simulink model "MPC_Controller"  (R2019b)
settings: Solver=VariableStepAuto  StartTime=0.0  StopTime=simStopTime  RelTol=1e-3
values from neighbouring files (symbols this model uses):
  curvatures = [curvatures; mean([lb.Curvature])]    [helperCreateReferencePath.m]    (also in onStartup.m = evaluator.curvatures)
  directions = ones(size(speedProfile))    [ControllerScript.m]
  mass = 2500    [ControllerScript.m]
  refPoses = [refPoses; [egoVehicle.Position(1:2), egoVehicle.Yaw]]    [helperCreateReferencePath.m]
  s = getValuesToEstimate(Exp)    [parameterEstimation.m]
  speedProfile = sqrt(sum(speedVector.*speedVector,2))    [ControllerScript.m]    (also in extractTheData.m = evaluator.velocities)
  theta0 = refPoses(1, 3)    [helperCreateReferencePath.m]
  Ts = 0.1    [ControllerScript.m]
  VEH =     [VEH.mat]
  x0 = refPoses(1, 1)    [helperCreateReferencePath.m]
  y0 = refPoses(1, 2)    [helperCreateReferencePath.m]
undefined symbols (not defined in the file or in its folder): driving, speedVector
libraries: simulink x2, autolibshared x2, drivingscenarioandsensors x2, mpcadaslib x1, sim3dlib x1, sim3dautolib x1, vehdynlibviscommon x1
settings Model: EnablePacing=on  PacingRate=1000  OrderedModelArguments=off  Creator=alaa  LastModifiedBy=LapTime
settings DataIOCC: SaveOutput=off  SignalLogging=off  DSMLogging=off  SaveTime=off  OutputOption=AdditionalOutputTimes  OutputTimes=simStopTime  ReturnWorkspaceOutputsName=SDOSimTest_Log
settings DebuggingCC: AlgebraicLoopMsg=none  ArtificialAlgebraicLoopMsg=none  MaxConsecutiveZCsMsg=none  ParameterPrecisionLossMsg=none  OperatingPointInterfaceChecksumMismatchMsg=none

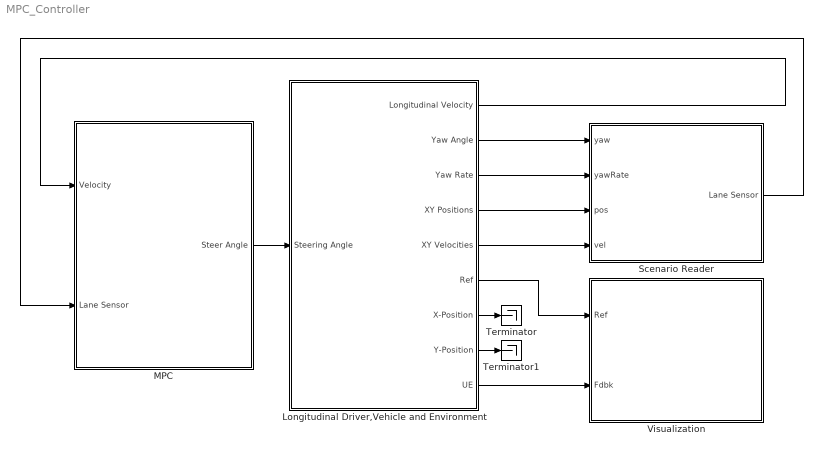
== system MPC_Controller ==
  Longitudinal Driver,Vehicle and Environment : Subsystem
  MPC : Subsystem
  Scenario Reader : Subsystem
  Terminator : Terminator
  Terminator1 : Terminator
  Visualization : Subsystem
  wires:
  Longitudinal Driver,Vehicle and Environment/1(Longitudinal Velocity) -> MPC/1(Velocity)
  Scenario Reader/1(Lane Sensor) -> MPC/2(Lane Sensor)
  Longitudinal Driver,Vehicle and Environment/5(XY Velocities) -> Scenario Reader/4(vel)
  Longitudinal Driver,Vehicle and Environment/2(Yaw Angle) -> Scenario Reader/1(yaw)
  Longitudinal Driver,Vehicle and Environment/3(Yaw Rate) -> Scenario Reader/2(yawRate)
  Longitudinal Driver,Vehicle and Environment/6(Ref) -> Visualization/1(Ref)
  Longitudinal Driver,Vehicle and Environment/4(XY Positions) -> Scenario Reader/3(pos)
  Longitudinal Driver,Vehicle and Environment/9("UE ") -> Visualization/2(Fdbk)
  Longitudinal Driver,Vehicle and Environment/7(X-Position) -> Terminator/1
  Longitudinal Driver,Vehicle and Environment/8(Y-Position) -> Terminator1/1
  MPC/1(Steer Angle) -> Longitudinal Driver,Vehicle and Environment/1(Steering Angle)

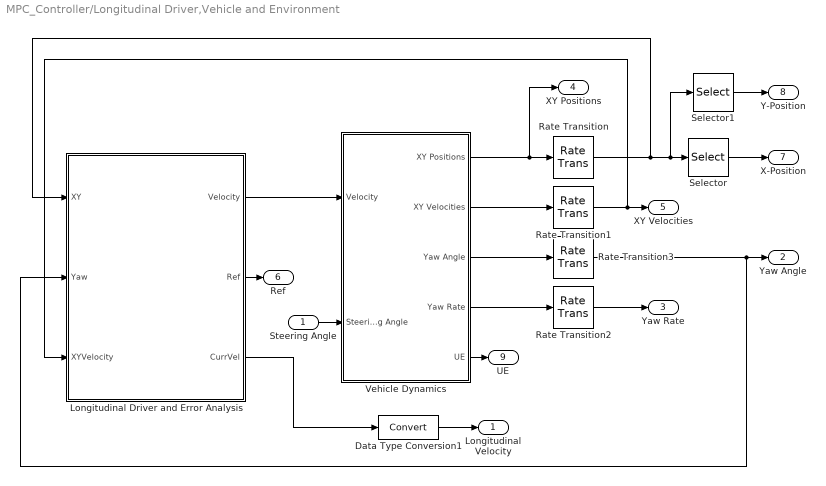
== system MPC_Controller/Longitudinal Driver,Vehicle and Environment ==
  Steering Angle : Inport  Unit=rad
  Data Type Conversion1 : DataTypeConversion
  Longitudinal Driver and Error Analysis : Subsystem
  Rate Transition : RateTransition  InitialCondition=[x0,y0]  OutPortSampleTime=Ts
  Rate Transition1 : RateTransition  InitialCondition=speedVector(1,1:2)  OutPortSampleTime=Ts
  Rate Transition2 : RateTransition  OutPortSampleTime=Ts
  Rate Transition3 : RateTransition  OutPortSampleTime=Ts
  Selector : Selector  InputPortWidth=2  IndexOptions=Index vector (dialog)  Indices=[1]  OutputSizes=1
  Selector1 : Selector  InputPortWidth=2  IndexOptions=Index vector (dialog)  Indices=[2]  OutputSizes=1
  Vehicle Dynamics : Subsystem  VariantControl=VariantVDBS
  Longitudinal Velocity : Outport  OutDataTypeStr=single  Unit=m/s  VectorParamsAs1DForOutWhenUnconnected=off
  Yaw Angle : Outport  Port=2
  Yaw Rate : Outport  Port=3
  XY Positions : Outport  Port=4
  XY Velocities : Outport  Port=5
  Ref : Outport  Port=6
  X-Position : Outport  Port=7
  Y-Position : Outport  Port=8
  "UE " : Outport  Port=9
  wires:
  Vehicle Dynamics/3(Yaw Angle) -> Rate Transition3/1
  Steering Angle/1 -> Vehicle Dynamics/2(Steering Angle)
  Data Type Conversion1/1 -> Longitudinal Velocity/1
  Longitudinal Driver and Error Analysis/3(CurrVel) -> Data Type Conversion1/1
  Longitudinal Driver and Error Analysis/1(Velocity) -> Vehicle Dynamics/1(Velocity)
  Selector/1 -> X-Position/1
  Selector1/1 -> Y-Position/1
  Vehicle Dynamics/2(XY Velocities) -> Rate Transition1/1
  Vehicle Dynamics/4(Yaw Rate) -> Rate Transition2/1
  Longitudinal Driver and Error Analysis/2(Ref) -> Ref/1
  Vehicle Dynamics/5("UE ") -> "UE "/1
  Rate Transition2/1 -> Yaw Rate/1
  Rate Transition1/1 -> XY Velocities/1, Longitudinal Driver and Error Analysis/3(XYVelocity)
  Rate Transition3/1 -> Yaw Angle/1, Longitudinal Driver and Error Analysis/2(Yaw)
  Vehicle Dynamics/1(XY Positions) -> XY Positions/1, Rate Transition/1
  Rate Transition/1 -> Selector1/1, Selector/1, Longitudinal Driver and Error Analysis/1(XY)

== system MPC_Controller/MPC ==
  Velocity : Inport
  Lane Sensor : Inport  Port=2
  Lane Center : Subsystem
  Lane Keeping Controller : mpcadaslib/Lane Keeping Assist System  ModelType=Use vehicle parameters  VehicleMass=mass  VehicleYawInertia=VEH.YawMomentInertia  LengthToFront=wheelbase-drear  LengthToRear=wheelbase-dfront  FrontTireStiffness=f_tire_stiff  RearTireStiffness=r_tire_stiff  EgoModelMatrixA=[-4.4021 ,-12.4603;1.3913,-5.1868]  EgoModelMatrixB=[24.1270;15.8609]  EgoModelMatrixC=[1,0;0,1]  InitialLongVel=speedProfile(1)  TransportLag=0  MinSteering=min_steer  umin_ext=off  MaxSteering=max_steer  umax_ext=off  Ts=Ts  PredictionHorizon=pred_Horizon  ControllerBehavior=aggressive  suboptimal=off  maxiter=10  datatypeopt=single  optmode=off  trackmode=off
      settings: SourceProductName=Model Predictive Control Toolbox  SourceProductBaseCode=MP
  Steer Angle : Outport
  wires:
  Lane Center/3(Heading Angle) -> Lane Keeping Controller/4
  Velocity/1 -> Lane Keeping Controller/2, Lane Center/2(Longitudinal Velocity)
  Lane Center/1(Previewed Curvature) -> Lane Keeping Controller/1
  Lane Center/2(Lateral Offset) -> Lane Keeping Controller/3
  Lane Sensor/1 -> Lane Center/1(Lane Detections)
  Lane Keeping Controller/1 -> Steer Angle/1

== system MPC_Controller/Scenario Reader ==
  yaw : Inport
  yawRate : Inport  Port=2
  pos : Inport  Port=3
  vel : Inport  Port=4
  Pack Ego Actor1 : MATLAB Function  TreatAsAtomicUnit=on
  Pack to Custom Sensor Data Format : Subsystem
  Scenario Reader : drivingscenarioandsensors/Scenario Reader  ScenarioSource=From workspace  ScenarioFileName=/home/alaa/Downloads/race-track-optimization/inc/controller/ankit.mat  ScenarioVariableName=scenario  OutputCoordinateSystem=Vehicle coordinates  EgoVehicleSource=Input port  EgoVehicleActorID=1  SampleTime=Ts  LaneBoundaryOutput=Ego vehicle lane boundaries  LaneBoundaryDistance=0:0.5:60  LaneBoundaryLocation=Inner edge of lane markings  BusNameSource=Auto  BusName=BusActors1Actors  BusName2Source=Auto  BusName2=BusLaneBoundaries  SimulateUsing=Interpreted execution
      settings: SourceProductName=Automated Driving Toolbox
  Terminator : Terminator
  Vision Detection Generator : drivingscenarioandsensors/Vision Detection Generator  SensorIndex=1  DetectorOutput=Lanes only  UpdateInterval=0.1  LaneUpdateInterval=0.1  SensorLocation=[ 1.9, 0 ]  Height=1.1  Yaw=0  Pitch=1  Roll=0  BusNameSource=Auto  BusName=BusObjectDetections  BusName2Source=Auto  BusName2=BusVision  MaxNumDetectionsSource=Property  MaxNumDetections=50  MaxNumLanesSource=Property  MaxNumLanes=2  DetectionCoordinates=Ego Cartesian  SimulateUsing=Interpreted execution  MaxRange=150  BoundingBoxAccuracy=5  ProcessNoiseIntensity=5  MaxSpeed=50  MaxAllowedOcclusion=0.5  MinObjectImageSize=[ 15, 15 ]  DetectionProbability=0.9  FalsePositivesPerImage=0.1  MinLaneImageSize=[ 20, 3 ]  LaneBoundaryAccuracy=3  HasNoise=on  InitialSeedSource=Repeatable  InitialSeed=0  UsedSeed=driving.internal.SimulinkUtilities.seedManager(gcb)  ActorProfilesSource=Parameters  ActorProfilesParameters=driving.internal.ActorProfilesParameters  ActorProfilesExpression=struct( 'ClassID', 0, 'Length', 4.7, 'Width', 1.8, 'Height', 1.4, 'OriginOffset', [ -1.35, 0, 0 ] )  Intrinsics=driving.internal.cameraIntrinsics
      settings: SourceProductName=Automated Driving Toolbox
  Lane Sensor : Outport
  wires:
  Pack Ego Actor1/1(a) -> Scenario Reader/1
  pos/1 -> Pack Ego Actor1/1(pos)
  Pack to Custom Sensor Data Format/1(Out) -> Lane Sensor/1
  Scenario Reader/2 -> Vision Detection Generator/1
  yaw/1 -> Pack Ego Actor1/3(yaw)
  Scenario Reader/1 -> Terminator/1
  Vision Detection Generator/1 -> Pack to Custom Sensor Data Format/1(In)
  vel/1 -> Pack Ego Actor1/2(vel)
  yawRate/1 -> Pack Ego Actor1/4(yawRate)

== system MPC_Controller/Visualization ==
  Ref : Inport
  Fdbk : Inport  Port=2
  Bus Selector : BusSelector  OutputSignals=InertFrm.Cg.Disp.X,InertFrm.Cg.Disp.Y,InertFrm.Cg.Vel.Xdot,InertFrm.Cg.Vel.Ydot
  Bus Selector1 : BusSelector  OutputSignals=InertFrm.Cg.Ang.phi,InertFrm.Cg.Ang.theta,InertFrm.Cg.Ang.psi  OutputAsBus=on
  Bus Selector5 : BusSelector  OutputSignals=BdyFrm.FrntAxl.Steer.WhlAngFR,BdyFrm.FrntAxl.Steer.WhlAngFL,BdyFrm.RearAxl.Steer.WhlAngRR,BdyFrm.RearAxl.Steer.WhlAngRL  OutputAsBus=on
  Bus to Vector1 : BusToVector
  Bus to Vector2 : BusToVector
  Mux : Mux  Inputs=2
  Mux1 : Mux  Inputs=2
  UE : Subsystem  Commented=on
  Visualization : Subsystem
  wires:
  Mux/1 -> Visualization/1(position)
  Mux1/1 -> Visualization/2(Velocity)
  Bus to Vector1/1 -> Visualization/5(WhlAng)
  Ref/1 -> Visualization/3(Ref)
  Bus to Vector2/1 -> Visualization/4(InertAng)
  Bus Selector/3 -> Mux1/1  "<Xdot>"
  Bus Selector/4 -> Mux1/2  "<Ydot>"
  Bus Selector/2 -> Mux/2  "<Y>"
  Bus Selector/1 -> Mux/1  "<X>"
  Fdbk/1 -> UE/1(VehFdbk), Bus Selector5/1, Bus Selector1/1, Bus Selector/1
  Bus Selector5/1 -> Bus to Vector1/1
  Bus Selector1/1 -> Bus to Vector2/1

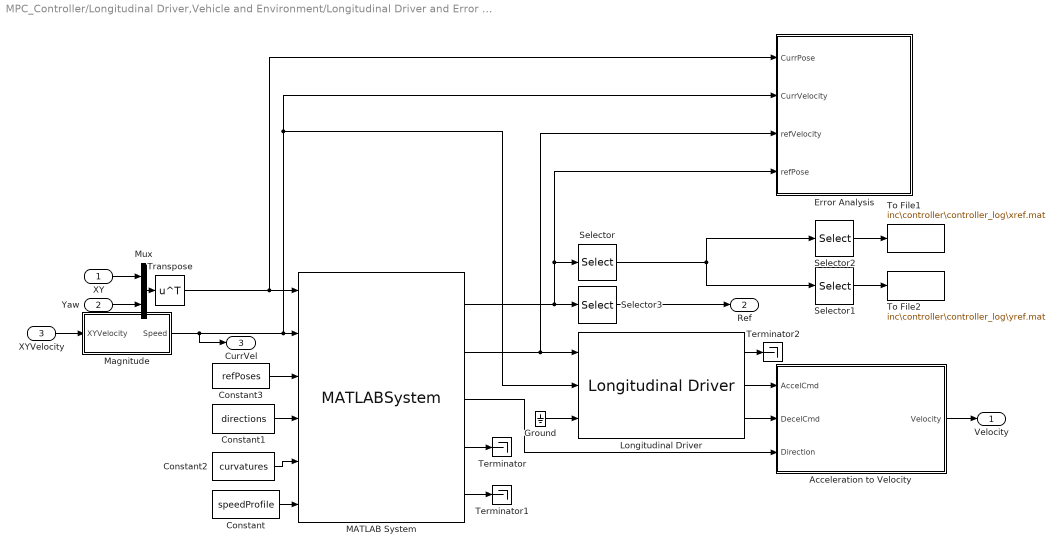
== system MPC_Controller/Longitudinal Driver,Vehicle and Environment/Longitudinal Driver and Error Analysis ==
  XY : Inport
  Yaw : Inport  Port=2
  XYVelocity : Inport  Port=3
  Acceleration to Velocity : Subsystem  TreatAsAtomicUnit=on
  Constant : Constant  Value=speedProfile  SampleTime=Ts
  Constant1 : Constant  Value=directions  SampleTime=Ts
  Constant2 : Constant  Value=curvatures  SampleTime=Ts
  Constant3 : Constant  Value=refPoses  SampleTime=Ts
  Error Analysis : Subsystem
  Ground : Ground
  Longitudinal Driver : autolibshared/Longitudinal Driver  cntrlType=Predictive  shftType=None  velUnits=m/s  gearOut=off  Kp=5  Ki=5  Kff=.1  Kg=0  VehVelVec=[0 100]  KffVec=[.1 .1]  KpVec=[10 10]  KiVec=[5 5]  KgVec=[0 0]  m=mass  Kpt=3000  tau=0.01  L=5  aR=200  bR=2.5  cR=VEH.DragCoefficient  g=9.81  vnom=5  Kaw=1  tauerr=.01  tauPt=2  GearInit=0  tShift=.1  pdlVec=[0.1 0.4 0.5 0.9]  upShftTbl=[-1 12.9375 26.4375 39.9375 51.18749999999999 62.4375 72.84375 83.25;-1 16.3125 29.8125 43.3125 54.5624 65.8125 76.78125 87.75;-1 19.6875 33.1875 46.68749999999999 57.9375 69.1875 80.71875 92.25;-1 33 52.5 77.25 100.5 138.75 161.875 185]  dwnShftTbl=[1 9.5625 23.0625 36.5625 47.8125 59.0625 68.90625 78.75;1 12.9375 26.4375 39.9375 51.18749999999999 62.4375 72.84375 83.25;1 16.3125 29.8125 43.3125 54.562499 65.8125 76.78125 87.75;1 19.6875 33.1875 46.68749999999999 57.9375 69.1875 80.71875 92.25]  tClutch=.5  tRev=.5  tPark=120  aMode=2  UpGearVec="[0  1  2  3  4  5  6  7]"  DownGearVec="[1  2  3  4  5  6  7  8]"
      settings: SourceProductName=Powertrain Blockset  SourceProductBaseCode=PW
  MATLAB System : MATLABSystem  System=HelperPathAnalyzer  Wheelbase=wheelbase  HasResetOutput=on  SimulateUsing=Interpreted execution
      mask Type: HelperPathAnalyzer
      mask Display:
      | disp(['Helper' char(10) 'Path' char(10) 'Analyzer']);
      | port_label('input',1,'CurrPose');
      | port_label('input',2,'CurrVelocity');
      | port_label('input',3,'RefPoses');
      | port_label('input',4,'Directions');
      | port_label('input',5,'Curvatures');
      | port_label('input',6,'SpeedProfile');
      | port_label('output',1,'RefPose');
      | port_label('output',2,'RefVelocity');
      | port_label('output',3,'Direction');
      | port_label('output',4,'Curvature');
      | port_label('output',5,'Reset');
  Magnitude : Subsystem
  Mux : Mux  Inputs=2
  Selector : Selector  InputPortWidth=3  IndexOptions=Index vector (dialog)  Indices=[1 2]  OutputSizes=1
  Selector1 : Selector  InputPortWidth=2  IndexOptions=Index vector (dialog)  Indices=[2]  OutputSizes=1
  Selector2 : Selector  InputPortWidth=2  IndexOptions=Index vector (dialog)  Indices=[1]  OutputSizes=1
  Selector3 : Selector  InputPortWidth=3  IndexOptions=Index vector (dialog)  Indices=[1 2]  OutputSizes=1
  Terminator : Terminator
  Terminator1 : Terminator
  Terminator2 : Terminator
  To File1 : ToFile  Filename=inc\controller\controller_log\xref.mat  MatrixName=xref
  To File2 : ToFile  Filename=inc\controller\controller_log\yref.mat  MatrixName=yref
  Transpose : Math  Operator=transpose  SignedPower=off  SaturateOnIntegerOverflow=on
  Velocity : Outport
  Ref : Outport  Port=2
  CurrVel : Outport  Port=3
  wires:
  MATLAB System/2 -> Error Analysis/3(refVelocity), Longitudinal Driver/1
  Constant2/1 -> MATLAB System/5
  Mux/1 -> Transpose/1
  Acceleration to Velocity/1(Velocity) -> Velocity/1
  Constant1/1 -> MATLAB System/4
  Constant/1 -> MATLAB System/6
  XY/1 -> Mux/1
  Selector/1 -> Selector2/1, Selector1/1
  MATLAB System/3 -> Acceleration to Velocity/3(Direction)
  Magnitude/1(Speed) -> CurrVel/1, Error Analysis/2(CurrVelocity), Longitudinal Driver/2, MATLAB System/2
  XYVelocity/1 -> Magnitude/1(XYVelocity)
  Yaw/1 -> Mux/2
  Longitudinal Driver/3 -> Acceleration to Velocity/2(DecelCmd)
  Longitudinal Driver/2 -> Acceleration to Velocity/1(AccelCmd)
  Selector2/1 -> To File1/1
  Selector1/1 -> To File2/1
  Constant3/1 -> MATLAB System/3
  MATLAB System/1 -> Selector3/1, Selector/1, Error Analysis/4(refPose)
  MATLAB System/5 -> Terminator1/1
  MATLAB System/4 -> Terminator/1
  Longitudinal Driver/1 -> Terminator2/1
  Ground/1 -> Longitudinal Driver/3
  Selector3/1 -> Ref/1
  Transpose/1 -> MATLAB System/1, Error Analysis/1(CurrPose)

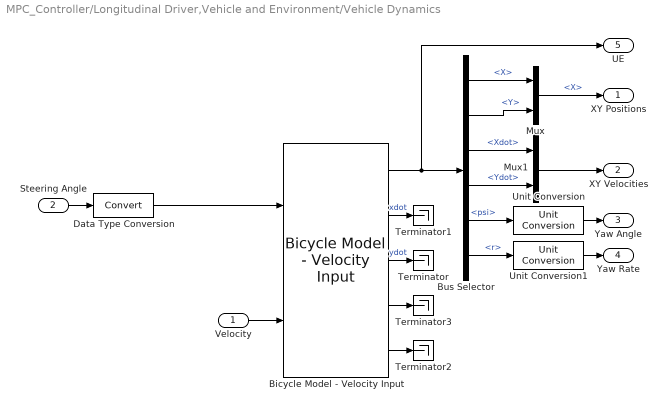
== system MPC_Controller/Longitudinal Driver,Vehicle and Environment/Vehicle Dynamics ==
  Velocity : Inport
  Steering Angle : Inport  Port=2
  Bicycle Model - Velocity Input : autolibshared/Bicycle Model - Velocity Input  trackMode=Single (bicycle)  inputMode=External longitudinal forces  frontSteerMode=on  rearSteerMode=off  windMode=off  muMode=off  extFMode=off  extMMode=off  aMode=3  NF=2  NR=2  m=mass  a=wheelbase-drear  b=wheelbase-dfront  h=h  X_o=x0  xdot_o=0  CalphaMode=off  sigmaMode=on  w=[1.4,1.4]  Cy_f=f_tire_stiff  Cy_r=r_tire_stiff  sigma_f=.1  sigma_r=.1  alpha_f_brk=[-.1 .1]  Cy_f_data=[-9e3 9e3]  alpha_r_brk=[-.1 .1]  Cy_r_data=[-9e3 9e3]  Y_o=y0  ydot_o=speedVector(1,2)  Izz=VEH.YawMomentInertia  psi_o=theta0*pi/180  r_o=0  Af=VEH.FrontalArea  Cd=VEH.DragCoefficient  Cl=0.1  Cpm=.1  beta_w=[0:0.01:0.3]  Cs=[0:0.03:0.9]  Cym=[0:0.01:0.3]  Pabs=101325  Tair=273  g=9.81  mu=mu  xdot_tol=.01  Fznom=5000  Fxtire_sat=1e6  Fytire_sat=1e6  longOff=0  latOff=0  vertOff=0
      settings: SourceProductName=Powertrain Blockset  SourceProductBaseCode=PW
  Bus Selector : BusSelector  OutputSignals=InertFrm.Cg.Disp.X,InertFrm.Cg.Disp.Y,InertFrm.Cg.Vel.Xdot,InertFrm.Cg.Vel.Ydot,InertFrm.Cg.Ang.psi,BdyFrm.Cg.AngVel.r
  Data Type Conversion : DataTypeConversion
  Mux : Mux  Inputs=2
  Mux1 : Mux  Inputs=2
  Terminator{,1..3} (4 alike) : Terminator
  Unit Conversion : UnitConversion  OutputType=Inherit: Inherit via back propagation
  Unit Conversion1 : UnitConversion  OutputType=Inherit: Inherit via back propagation
  XY Positions : Outport  Unit=m  VectorParamsAs1DForOutWhenUnconnected=off
  XY Velocities : Outport  Port=2  Unit=m/s  VectorParamsAs1DForOutWhenUnconnected=off
  Yaw Angle : Outport  Port=3  Unit=deg  VectorParamsAs1DForOutWhenUnconnected=off
  Yaw Rate : Outport  Port=4  Unit=degree/s  VectorParamsAs1DForOutWhenUnconnected=off
  "UE " : Outport  Port=5
  wires:
  Mux1/1 -> XY Velocities/1
  Unit Conversion1/1 -> Yaw Rate/1
  Unit Conversion/1 -> Yaw Angle/1
  Bus Selector/1 -> Mux/1  "<X>"
  Bus Selector/2 -> Mux/2  "<Y>"
  Bus Selector/4 -> Mux1/2  "<Ydot>"
  Bus Selector/3 -> Mux1/1  "<Xdot>"
  Steering Angle/1 -> Data Type Conversion/1
  Data Type Conversion/1 -> Bicycle Model - Velocity Input/1
  Velocity/1 -> Bicycle Model - Velocity Input/2
  Mux/1 -> XY Positions/1  "<X>"
  Bicycle Model - Velocity Input/1 -> "UE "/1, Bus Selector/1
  Bicycle Model - Velocity Input/2 -> Terminator1/1  "xdot"
  Bicycle Model - Velocity Input/3 -> Terminator/1  "ydot"
  Bus Selector/5 -> Unit Conversion/1  "<psi>"
  Bus Selector/6 -> Unit Conversion1/1  "<r>"
  Bicycle Model - Velocity Input/5 -> Terminator2/1
  Bicycle Model - Velocity Input/4 -> Terminator3/1

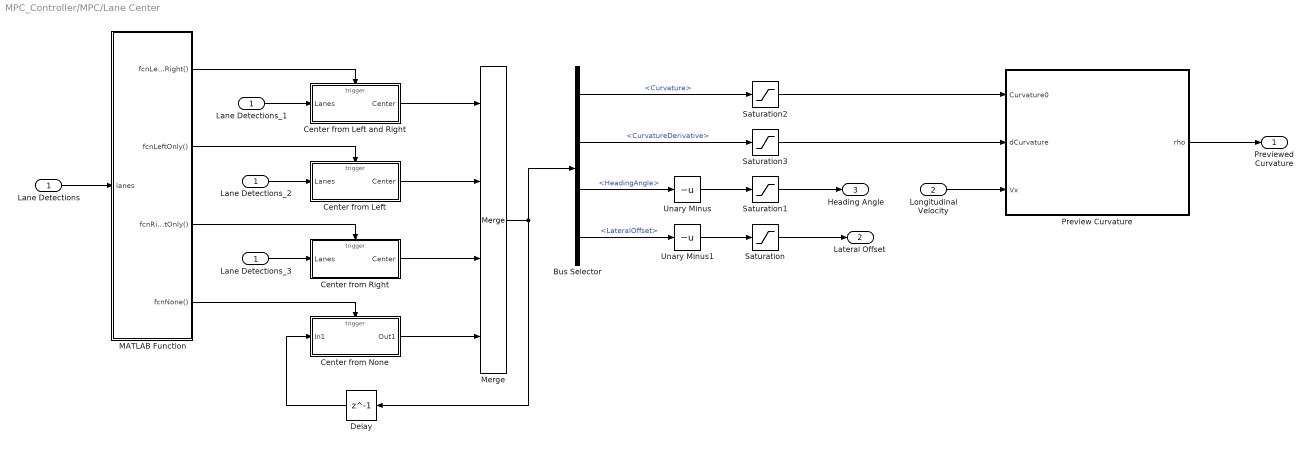
== system MPC_Controller/MPC/Lane Center ==
  Lane Detections : Inport
  Longitudinal Velocity : Inport  Port=2  OutDataTypeStr=single
  Bus Selector : BusSelector  OutputSignals=Curvature,CurvatureDerivative,HeadingAngle,LateralOffset
  Center from Left : Subsystem  TreatAsAtomicUnit=on
  Center from Left and Right : Subsystem  TreatAsAtomicUnit=on
  Center from None : Subsystem  TreatAsAtomicUnit=on
  Center from Right : Subsystem  TreatAsAtomicUnit=on
  Delay : Delay  DelayLength=1
  Lane Detections_1 : InportShadow
  Lane Detections_2 : InportShadow
  Lane Detections_3 : InportShadow
  MATLAB Function : MATLAB Function  TreatAsAtomicUnit=on
  Merge : Merge  Inputs=4
  Preview Curvature : MATLAB Function  TreatAsAtomicUnit=on  SystemSampleTime=Ts
  Saturation : Saturate
  Saturation1 : Saturate  UpperLimit=0.6  LowerLimit=-0.6
  Saturation2 : Saturate  UpperLimit=0.15  LowerLimit=-0.15
  Saturation3 : Saturate  UpperLimit=0.06  LowerLimit=-0.06
  Unary Minus : UnaryMinus
  Unary Minus1 : UnaryMinus
  Previewed Curvature : Outport  VectorParamsAs1DForOutWhenUnconnected=off
  Lateral Offset : Outport  Port=2  VectorParamsAs1DForOutWhenUnconnected=off
  Heading Angle : Outport  Port=3  VectorParamsAs1DForOutWhenUnconnected=off
  wires:
  Saturation2/1 -> Preview Curvature/1(Curvature0)
  Bus Selector/2 -> Saturation3/1  "<CurvatureDerivative>"
  Longitudinal Velocity/1 -> Preview Curvature/3(Vx)
  Merge/1 -> Delay/1, Bus Selector/1
  Center from Left and Right/1(Center) -> Merge/1
  Unary Minus/1 -> Saturation1/1
  Center from None/1(Out1) -> Merge/4
  MATLAB Function/3(fcnRightOnly()) -> Center from Right/Trigger
  Lane Detections_2/1 -> Center from Left/1(Lanes)
  MATLAB Function/1(fcnLeftAndRight()) -> Center from Left and Right/Trigger
  MATLAB Function/2(fcnLeftOnly()) -> Center from Left/Trigger
  Preview Curvature/1(rho) -> Previewed Curvature/1
  Saturation/1 -> Lateral Offset/1
  Lane Detections_1/1 -> Center from Left and Right/1(Lanes)
  Lane Detections/1 -> MATLAB Function/1(lanes)
  Bus Selector/1 -> Saturation2/1  "<Curvature>"
  Center from Right/1(Center) -> Merge/3
  Saturation1/1 -> Heading Angle/1
  Saturation3/1 -> Preview Curvature/2(dCurvature)
  Center from Left/1(Center) -> Merge/2
  Bus Selector/4 -> Unary Minus1/1  "<LateralOffset>"
  Delay/1 -> Center from None/1(In1)
  Unary Minus1/1 -> Saturation/1
  Bus Selector/3 -> Unary Minus/1  "<HeadingAngle>"
  Lane Detections_3/1 -> Center from Right/1(Lanes)
  MATLAB Function/4(fcnNone()) -> Center from None/Trigger

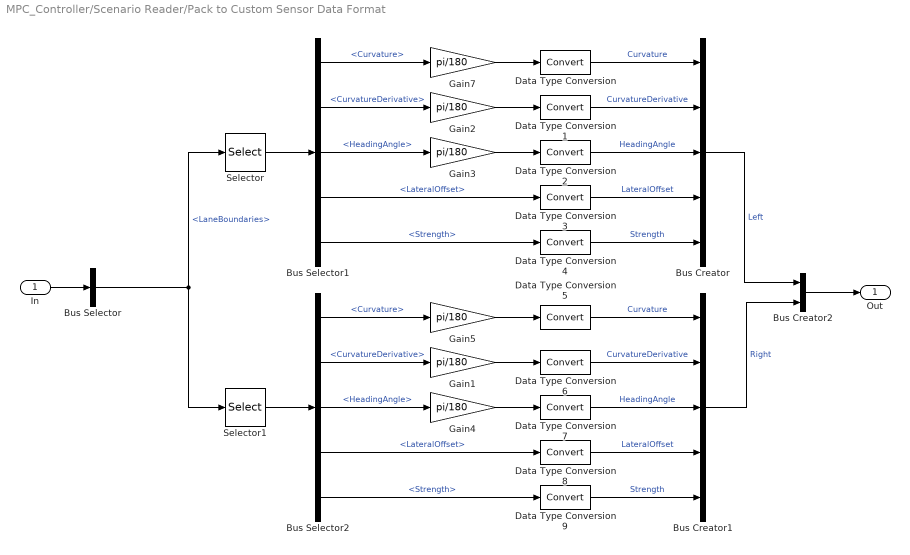
== system MPC_Controller/Scenario Reader/Pack to Custom Sensor Data Format ==
  In : Inport
  Bus Creator : BusCreator  Inputs=5  OutDataTypeStr=Bus: LaneSensorBoundaries
      settings: InheritFromInputs=off
  Bus Creator1 : BusCreator  Inputs=5  OutDataTypeStr=Bus: LaneSensorBoundaries
  Bus Creator2 : BusCreator  Inputs=2  OutDataTypeStr=Bus: LaneSensor
  Bus Selector : BusSelector  OutputSignals=LaneBoundaries
  Bus Selector1 : BusSelector  OutputSignals=Curvature,CurvatureDerivative,HeadingAngle,LateralOffset,Strength
  Bus Selector2 : BusSelector  OutputSignals=Curvature,CurvatureDerivative,HeadingAngle,LateralOffset,Strength
  Data Type Conversion{,1..9} (10 alike) : DataTypeConversion
  Gain{1..5,7} (6 alike) : Gain  Gain=pi/180
  Selector : Selector  InputPortWidth=2  IndexOptions=Index vector (dialog)  Indices=1  OutputSizes=1
  Selector1 : Selector  InputPortWidth=2  IndexOptions=Index vector (dialog)  Indices=2  OutputSizes=1
  Out : Outport  VectorParamsAs1DForOutWhenUnconnected=off
  wires:
  In/1 -> Bus Selector/1
  Bus Selector/1 -> Selector/1, Selector1/1  "<LaneBoundaries>"
  Selector/1 -> Bus Selector1/1
  Bus Selector1/2 -> Gain2/1  "<CurvatureDerivative>"
  Bus Selector1/1 -> Gain7/1  "<Curvature>"
  Bus Selector1/3 -> Gain3/1  "<HeadingAngle>"
  Gain7/1 -> Data Type Conversion/1
  Gain2/1 -> Data Type Conversion1/1
  Gain3/1 -> Data Type Conversion2/1
  Bus Selector1/4 -> Data Type Conversion3/1  "<LateralOffset>"
  Bus Selector1/5 -> Data Type Conversion4/1  "<Strength>"
  Data Type Conversion/1 -> Bus Creator/1  "Curvature"
  Data Type Conversion1/1 -> Bus Creator/2  "CurvatureDerivative"
  Data Type Conversion2/1 -> Bus Creator/3  "HeadingAngle"
  Data Type Conversion3/1 -> Bus Creator/4  "LateralOffset"
  Data Type Conversion4/1 -> Bus Creator/5  "Strength"
  Data Type Conversion9/1 -> Bus Creator1/5  "Strength"
  Data Type Conversion6/1 -> Bus Creator1/2  "CurvatureDerivative"
  Data Type Conversion7/1 -> Bus Creator1/3  "HeadingAngle"
  Data Type Conversion8/1 -> Bus Creator1/4  "LateralOffset"
  Data Type Conversion5/1 -> Bus Creator1/1  "Curvature"
  Bus Selector2/1 -> Gain5/1  "<Curvature>"
  Selector1/1 -> Bus Selector2/1
  Bus Selector2/4 -> Data Type Conversion8/1  "<LateralOffset>"
  Bus Selector2/5 -> Data Type Conversion9/1  "<Strength>"
  Bus Selector2/2 -> Gain1/1  "<CurvatureDerivative>"
  Gain4/1 -> Data Type Conversion7/1
  Gain5/1 -> Data Type Conversion5/1
  Gain1/1 -> Data Type Conversion6/1
  Bus Selector2/3 -> Gain4/1  "<HeadingAngle>"
  Bus Creator2/1 -> Out/1
  Bus Creator/1 -> Bus Creator2/1  "Left"
  Bus Creator1/1 -> Bus Creator2/2  "Right"

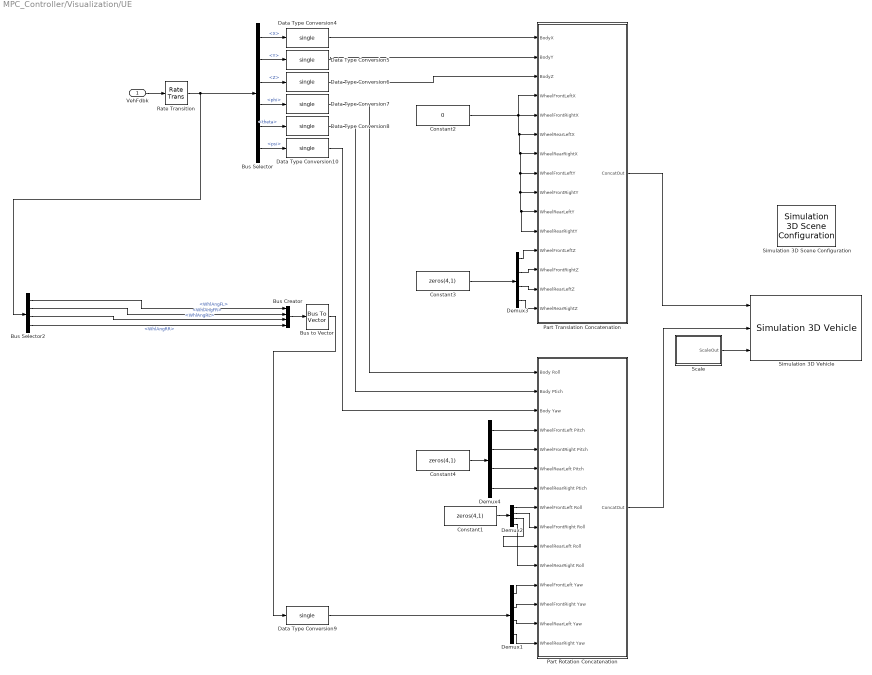
== system MPC_Controller/Visualization/UE ==
  VehFdbk : Inport
  Bus Creator : BusCreator  Inputs=4
  Bus Selector : BusSelector  OutputSignals=InertFrm.Cg.Disp.X,InertFrm.Cg.Disp.Y,InertFrm.Cg.Disp.Z,InertFrm.Cg.Ang.phi,InertFrm.Cg.Ang.theta,InertFrm.Cg.Ang.psi
  Bus Selector2 : BusSelector  OutputSignals=BdyFrm.FrntAxl.Steer.WhlAngFL,BdyFrm.FrntAxl.Steer.WhlAngFR,BdyFrm.RearAxl.Steer.WhlAngRL,BdyFrm.RearAxl.Steer.WhlAngRR
  Bus to Vector : BusToVector
  Constant1 : Constant  Value=zeros(4,1)  OutDataTypeStr=single
  Constant2 : Constant  Value=0  OutDataTypeStr=single
  Constant3 : Constant  Value=zeros(4,1)  OutDataTypeStr=single
  Constant4 : Constant  Value=zeros(4,1)  OutDataTypeStr=single
  Data Type Conversion{4..10} (7 alike) : DataTypeConversion  OutDataTypeStr=single
  Demux{1..4} (4 alike) : Demux
  Part Rotation Concatenation : Subsystem
  Part Translation Concatenation : Subsystem
  Rate Transition : RateTransition  OutPortSampleTime=Ts
  Scale : Subsystem
  Simulation 3D Scene Configuration : sim3dlib/Simulation 3D Scene Configuration  Priority=0  SceneDesc=US city block  vehTagList={'Scene Origin';'SimulinkVehicle1'}  vehTag=SimulinkVehicle1  OpVisEn=off  Ts=Ts  ProjectFormat=Executable  ProjectName=VehicleSimulation.exe  sensorTag=MainCamera1  sensorId=1  sensorName=MainCamera1  mountLoc=Origin  offsetFlag=off  tmountOffset=[0, 0, 0]  rmountOffset=[0, 0, 0]  HorizontalResolution=1280  VerticalResolution=720  HorizontalFOV=60  mountPoint=[0 0 0]  mountOrientation=[0 0 0]  aMode=aMode  ID=1
      settings: SourceProductName=Automated Driving Toolbox  SourceProductBaseCode=DR
  Simulation 3D Vehicle : sim3dautolib/Simulation 3D Vehicle  Priority=-1  PassVehMesh=Muscle car  VehColor=Red  ActorName=SimulinkVehicle1  Translation=[x0 y0 0; 0 0 0; 0 0 0; 0 0 0; 0 0 0]  Rotation=[0 0 theta0; 0 0 0; 0 0 0; 0 0 0; 0 0 0]  Scale=ones( 5, 3 )  SampleTime=Ts  ActorType=SimulinkVehicle  ID=1  aMode=2  ActorTag=SimulinkVehicle1
      settings: SourceProductName=Automated Driving Toolbox  SourceProductBaseCode=DR
  wires:
  Demux2/2 -> Part Rotation Concatenation/9(WheelFrontRight Roll)
  Bus Selector/5 -> Data Type Conversion8/1  "<theta>"
  Demux2/1 -> Part Rotation Concatenation/8(WheelFrontLeft Roll)
  Data Type Conversion6/1 -> Part Translation Concatenation/3(BodyZ)
  Demux1/4 -> Part Rotation Concatenation/15(WheelRearRight Yaw)
  Bus Selector/3 -> Data Type Conversion6/1  "<Z>"
  Data Type Conversion9/1 -> Demux1/1
  Data Type Conversion7/1 -> Part Rotation Concatenation/1(Body Roll)
  Rate Transition/1 -> Bus Selector/1, Bus Selector2/1
  Bus Selector/6 -> Data Type Conversion10/1  "<psi>"
  Demux2/3 -> Part Rotation Concatenation/10(WheelRearLeft Roll)
  Data Type Conversion4/1 -> Part Translation Concatenation/1(BodyX)
  Constant2/1 -> Part Translation Concatenation/5(WheelFrontRightX), Part Translation Concatenation/6(WheelRearLeftX), Part Translation Concatenation/7(WheelRearRightX), Part Translation Concatenation/8(WheelFrontLeftY), Part Translation Concatenation/9(WheelFrontRightY), Part Translation Concatenation/10(WheelRearLeftY), Part Translation Concatenation/11(WheelRearRightY), Part Translation Concatenation/4(WheelFrontLeftX)
  Part Rotation Concatenation/1(ConcatOut) -> Simulation 3D Vehicle/2
  Demux3/2 -> Part Translation Concatenation/13(WheelFrontRightZ)
  Demux1/2 -> Part Rotation Concatenation/13(WheelFrontRight Yaw)
  Part Translation Concatenation/1(ConcatOut) -> Simulation 3D Vehicle/1
  Constant1/1 -> Demux2/1
  Bus Selector/2 -> Data Type Conversion5/1  "<Y>"
  Data Type Conversion10/1 -> Part Rotation Concatenation/3(Body Yaw)
  Bus Selector/1 -> Data Type Conversion4/1  "<X>"
  Demux3/3 -> Part Translation Concatenation/14(WheelRearLeftZ)
  Data Type Conversion5/1 -> Part Translation Concatenation/2(BodyY)
  Demux3/4 -> Part Translation Concatenation/15(WheelRearRightZ)
  Demux1/1 -> Part Rotation Concatenation/12(WheelFrontLeft Yaw)
  Data Type Conversion8/1 -> Part Rotation Concatenation/2(Body Ptich)
  Demux2/4 -> Part Rotation Concatenation/11(WheelRearRight Roll)
  Demux3/1 -> Part Translation Concatenation/12(WheelFrontLeftZ)
  Demux1/3 -> Part Rotation Concatenation/14(WheelRearLeft Yaw)
  Scale/1(ScaleOut) -> Simulation 3D Vehicle/3
  VehFdbk/1 -> Rate Transition/1
  Bus Selector/4 -> Data Type Conversion7/1  "<phi>"
  Bus Creator/1 -> Bus to Vector/1
  Bus Selector2/1 -> Bus Creator/1  "<WhlAngFL>"
  Bus Selector2/2 -> Bus Creator/2  "<WhlAngFR>"
  Bus Selector2/3 -> Bus Creator/3  "<WhlAngRL>"
  Bus Selector2/4 -> Bus Creator/4  "<WhlAngRR>"
  Bus to Vector/1 -> Data Type Conversion9/1
  Constant3/1 -> Demux3/1
  Constant4/1 -> Demux4/1
  Demux4/1 -> Part Rotation Concatenation/4(WheelFrontLeft Pitch)
  Demux4/2 -> Part Rotation Concatenation/5(WheelFrontRight Pitch)
  Demux4/3 -> Part Rotation Concatenation/6(WheelRearLeft Pitch)
  Demux4/4 -> Part Rotation Concatenation/7(WheelRearRight Ptich)

== system MPC_Controller/Visualization/Visualization ==
  position : Inport
  Velocity : Inport  Port=2
  Ref : Inport  Port=3
  InertAng : Inport  Port=4
  WhlAng : Inport  Port=5
  Ground1 : Ground
  Ground2 : Ground
  Mux1 : Mux  Inputs=2
  Mux2 : Mux  Inputs=2
  Vehicle XY Plotter : Subsystem  mask(Vehicle XY Plotter){a=wheelbase-drear, b=wheelbase-dfront, w=VEH.TrackWidth, figBorder=10, bufferSize=1024, extRef=on, pltDT=Ts}
      mask prompts: a "Distance to front axle from CG, a [m]:"; b "Distance to rear axle from CG, b [m]:"; w "Track width, w [m]:"; figBorder "Distance to figure borders, figBorder [m]:"; bufferSize "Path buffer sampe size, bufferSize []:"; extRef "Plot path reference, extRef"; pltDT "Plot update rate, pltDT [s]:"
      mask help:
      | This block will display a MATLAB figure which indicates the vehicle path, current position and heading velocity.
      | An optional path reference is also provided.
      mask init:
      | if autoblkschecksimstopped(gcb)
      |     PortName = 'RefXYZ';
      |     InportOption  = {'built-in/Ground', [PortName, ' Ground'];...
      |         'built-in/Inport',PortName };
      |     if ~strcmp(get_param(gcb,'extRef'),'on')
      |         NewBlkHdl = autoblksreplaceblock(gcb, InportOption, 1);
      |         set_param(NewBlkHdl, 'ShowName', 'off');
      |     else
      |         autoblksreplaceblock(gcb, InportOption, 2);
      |     end
      | end
      mask TypeOptions a: Vehicle XY Plotter/a
      mask TypeOptions b: Vehicle XY Plotter/b
      mask TypeOptions w: Vehicle XY Plotter/w
      mask TypeOptions figBorder: Vehicle XY Plotter/figBorder
      mask TypeOptions bufferSize: Vehicle XY Plotter/bufferSize
  wires:
  InertAng/1 -> Vehicle XY Plotter/2(InertAng)
  position/1 -> Vehicle XY Plotter/1(InertXYZ)
  Ground1/1 -> Mux1/2
  WhlAng/1 -> Vehicle XY Plotter/4(WhlAng)
  Ref/1 -> Mux1/1
  Velocity/1 -> Mux2/1
  Ground2/1 -> Mux2/2
  Mux2/1 -> Vehicle XY Plotter/3(InertXdotYdotZdot)
  Mux1/1 -> Vehicle XY Plotter/5(RefXYZ)

== system MPC_Controller/Longitudinal Driver,Vehicle and Environment/Longitudinal Driver and Error Analysis/Acceleration to Velocity ==
  AccelCmd : Inport  PortDimensions=[1 1]
  DecelCmd : Inport  Port=2  PortDimensions=[1 1]
  Direction : Inport  Port=3
  AND : Logic  IconShape=distinctive  AllPortsSameDT=off  OutDataTypeStr=boolean
  Abs : Abs
  Add : Sum  Inputs=+-
  Compare To Zero : simulink/Logic and Bit Operations/Compare To Zero  relop=<=  OutDataTypeStr=boolean
  Compare To Zero1 : simulink/Logic and Bit Operations/Compare To Zero  relop=>  OutDataTypeStr=boolean
  Constant : Constant  Value=0.05
  Constant1 : Constant  Value=0  SampleTime=Ts
  Minus : Sum  Inputs=+-
  Product1 : Product
  Saturated integrator : Integrator  ExternalReset=either  LimitOutput=on  LowerSaturationLimit=0  AbsoluteTolerance=1e-3  ZeroCross=off
  Switch : Switch  Criteria=u2 > Threshold
  Unit Delay : UnitDelay  InitialCondition=speedProfile(1)  SampleTime=Ts  HasFrameUpgradeWarning=on
  Velocity : Outport  VectorParamsAs1DForOutWhenUnconnected=off
  wires:
  Direction/1 -> Product1/2, Saturated integrator/2
  AccelCmd/1 -> Add/1
  Add/1 -> Saturated integrator/1
  DecelCmd/1 -> Compare To Zero1/1, Add/2
  Unit Delay/1 -> Abs/1
  Abs/1 -> Minus/1
  Constant/1 -> Minus/2
  Minus/1 -> Compare To Zero/1
  Compare To Zero/1 -> AND/2
  Compare To Zero1/1 -> AND/1
  AND/1 -> Switch/2  "Reset velocity to zero"
  Switch/1 -> Velocity/1, Unit Delay/1
  Constant1/1 -> Switch/1
  Saturated integrator/1 -> Product1/1
  Product1/1 -> Switch/3

== system MPC_Controller/Longitudinal Driver,Vehicle and Environment/Longitudinal Driver and Error Analysis/Error Analysis ==
  CurrPose : Inport
  CurrVelocity : Inport  Port=2
  refVelocity : Inport  Port=3
  refPose : Inport  Port=4
  Divide : Product  Inputs=*/  SaturateOnIntegerOverflow=on  RndMeth=Zero
  Divide1 : Product  Inputs=*/  SaturateOnIntegerOverflow=on  RndMeth=Zero
  Scope1 : Scope
  Scope3 : Scope
  Sum : Sum  Inputs=|+-
  Sum1 : Sum  Inputs=|+-
  To File : ToFile  Filename=inc\controller\controller_log\positionerror  MatrixName=positionerror  SaveFormat=Timeseries
  To File2 : ToFile  Filename=inc\controller\controller_log\VelocityError  MatrixName=VelocityError  SaveFormat=Timeseries
  wires:
  CurrVelocity/1 -> Sum/2
  refVelocity/1 -> Divide/2, Sum/1
  Sum/1 -> Divide/1
  Divide/1 -> To File2/1, Scope1/1  "Velocity Error"
  Divide1/1 -> To File/1, Scope3/1  "Position Error"
  CurrPose/1 -> Sum1/2
  refPose/1 -> Divide1/2, Sum1/1
  Sum1/1 -> Divide1/1

== system MPC_Controller/Longitudinal Driver,Vehicle and Environment/Longitudinal Driver and Error Analysis/Magnitude ==
  XYVelocity : Inport
  Add1 : Sum
  Selector1 : Selector  InputPortWidth=2  IndexOptions=Index vector (dialog)  Indices=[2]  OutputSizes=1
  Selector2 : Selector  InputPortWidth=2  IndexOptions=Index vector (dialog)  Indices=[1]  OutputSizes=1
  Sqrt : Sqrt  SaturateOnIntegerOverflow=on
  Square : Math  Operator=square  SignedPower=off  SaturateOnIntegerOverflow=on
  Square1 : Math  Operator=square  SignedPower=off  SaturateOnIntegerOverflow=on
  Speed : Outport
  wires:
  Selector1/1 -> Square1/1
  Square/1 -> Add1/1
  Sqrt/1 -> Speed/1
  XYVelocity/1 -> Selector2/1, Selector1/1
  Add1/1 -> Sqrt/1
  Square1/1 -> Add1/2
  Selector2/1 -> Square/1

== system MPC_Controller/MPC/Lane Center/Center from Left ==
  note: Curvature
      | = 1 / ( 1 / (left curvature) – guard)
      | = left curvature / (1 – (left curvature) * guard).
  note: Center from Left
  note: Curvature Derivative
      | = D[ 1 / ( 1 / (left curvature) – guard)]
      | = left curvature derivative / (1 – (left curvature) * guard)^2.
  In Bus Element : Inport  PortName=Lanes  Element=Left.Curvature
  In Bus Element2 : Inport  PortName=Lanes  Element=Left.CurvatureDerivative
  In Bus Element4 : Inport  PortName=Lanes  Element=Left.HeadingAngle
  In Bus Element6 : Inport  PortName=Lanes  Element=Left.LateralOffset
  function : TriggerPort  TriggerType=function-call  VariantControl=Variant
  Bus Creator : BusCreator  Inputs=4
  Constant : Constant  OutDataTypeStr=Inherit: Inherit via back propagation
  Divide : Product  Inputs=*/
  Divide1 : Product  Inputs=*/
  Half Lane Width Estimate : Constant  Value=1.8  OutDataTypeStr=Inherit: Inherit via back propagation
  Half Lane Width Estimate1 : Constant  Value=1.8  OutDataTypeStr=Inherit: Inherit via back propagation
  Product : Product
  Product1 : Product
  Subtract : Sum  Inputs=+-
  Subtract1 : Sum  Inputs=+-
  Center : Outport  VectorParamsAs1DForOutWhenUnconnected=off
  wires:
  Bus Creator/1 -> Center/1
  Divide1/1 -> Bus Creator/2  "CurvatureDerivative"
  Divide/1 -> Bus Creator/1  "Curvature"
  In Bus Element4/1 -> Bus Creator/3  "HeadingAngle"
  Subtract1/1 -> Bus Creator/4  "LateralOffset"
  In Bus Element/1 -> Product/1, Divide/1  "Curvature"
  Subtract/1 -> Product1/2, Product1/1, Divide/2
  Half Lane Width Estimate/1 -> Product/2
  Constant/1 -> Subtract/1
  In Bus Element2/1 -> Divide1/1  "CurvatureDerivative"
  Product1/1 -> Divide1/2
  In Bus Element6/1 -> Subtract1/1  "LateralOffset"
  Half Lane Width Estimate1/1 -> Subtract1/2
  Product/1 -> Subtract/2

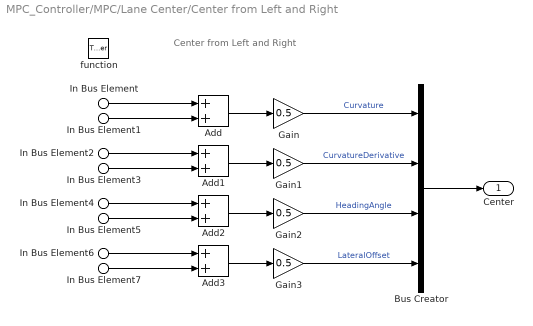
== system MPC_Controller/MPC/Lane Center/Center from Left and Right ==
  note: Center from Left and Right
  In Bus Element : Inport  PortName=Lanes  Element=Left.Curvature
  In Bus Element2 : Inport  PortName=Lanes  Element=Left.CurvatureDerivative
  In Bus Element4 : Inport  PortName=Lanes  Element=Left.HeadingAngle
  In Bus Element6 : Inport  PortName=Lanes  Element=Left.LateralOffset
  In Bus Element1 : Inport  PortName=Lanes  Element=Right.Curvature
  In Bus Element3 : Inport  PortName=Lanes  Element=Right.CurvatureDerivative
  In Bus Element5 : Inport  PortName=Lanes  Element=Right.HeadingAngle
  In Bus Element7 : Inport  PortName=Lanes  Element=Right.LateralOffset
  function : TriggerPort  TriggerType=function-call  VariantControl=Variant
  Add{,1..3} (4 alike) : Sum
  Bus Creator : BusCreator  Inputs=4
  Gain{,1..3} (4 alike) : Gain  Gain=0.5
  Center : Outport  VectorParamsAs1DForOutWhenUnconnected=off
  wires:
  Add/1 -> Gain/1
  Gain/1 -> Bus Creator/1  "Curvature"
  Add1/1 -> Gain1/1
  Gain1/1 -> Bus Creator/2  "CurvatureDerivative"
  Add2/1 -> Gain2/1
  Gain2/1 -> Bus Creator/3  "HeadingAngle"
  Add3/1 -> Gain3/1
  Gain3/1 -> Bus Creator/4  "LateralOffset"
  Bus Creator/1 -> Center/1
  In Bus Element/1 -> Add/1
  In Bus Element1/1 -> Add/2
  In Bus Element2/1 -> Add1/1
  In Bus Element3/1 -> Add1/2
  In Bus Element4/1 -> Add2/1
  In Bus Element5/1 -> Add2/2
  In Bus Element7/1 -> Add3/2
  In Bus Element6/1 -> Add3/1

== system MPC_Controller/MPC/Lane Center/Center from None ==
  In1 : Inport
  function : TriggerPort  TriggerType=function-call  VariantControl=Variant
  Out1 : Outport  VectorParamsAs1DForOutWhenUnconnected=off
  wires:
  In1/1 -> Out1/1

== system MPC_Controller/MPC/Lane Center/Center from Right ==
  note: Center from Right
  note: Curvature
      | = 1 / ( 1 / (right curvature) + guard)
      | = right curvature / (1 + (right curvature) * guard)
  note: Curvature Derivative
      | = D[ 1 / ( 1 / (right curvature) + guard)]
      | = right curvature derivative / (1 + (right curvature) * guard)^2
  In Bus Element : Inport  PortName=Lanes  Element=Right.Curvature
  In Bus Element2 : Inport  PortName=Lanes  Element=Right.CurvatureDerivative
  In Bus Element4 : Inport  PortName=Lanes  Element=Right.HeadingAngle
  In Bus Element6 : Inport  PortName=Lanes  Element=Right.LateralOffset
  function : TriggerPort  TriggerType=function-call  VariantControl=Variant
  Bus Creator : BusCreator  Inputs=4
  Constant : Constant  OutDataTypeStr=Inherit: Inherit via back propagation
  Divide : Product  Inputs=*/
  Divide1 : Product  Inputs=*/
  Half Lane Width Estimate : Constant  Value=1.8  OutDataTypeStr=Inherit: Inherit via back propagation
  Half Lane Width Estimate1 : Constant  Value=1.8  OutDataTypeStr=Inherit: Inherit via back propagation
  Product : Product
  Product1 : Product
  Subtract : Sum
  Subtract1 : Sum
  Center : Outport  VectorParamsAs1DForOutWhenUnconnected=off
  wires:
  In Bus Element2/1 -> Divide1/1  "CurvatureDerivative"
  Divide1/1 -> Bus Creator/2  "CurvatureDerivative"
  Product1/1 -> Divide1/2
  In Bus Element4/1 -> Bus Creator/3  "HeadingAngle"
  Half Lane Width Estimate1/1 -> Subtract1/2
  In Bus Element6/1 -> Subtract1/1  "LateralOffset"
  Divide/1 -> Bus Creator/1  "Curvature"
  Subtract1/1 -> Bus Creator/4  "LateralOffset"
  Bus Creator/1 -> Center/1
  In Bus Element/1 -> Product/1, Divide/1  "Curvature"
  Subtract/1 -> Product1/2, Product1/1, Divide/2
  Constant/1 -> Subtract/1
  Product/1 -> Subtract/2
  Half Lane Width Estimate/1 -> Product/2

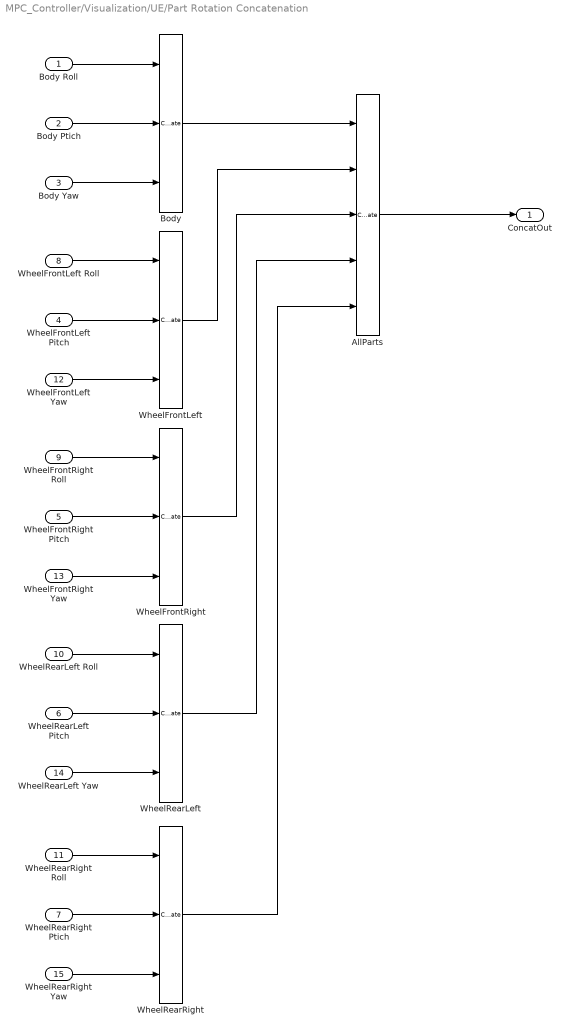
== system MPC_Controller/Visualization/UE/Part Rotation Concatenation ==
  Body Roll : Inport
  Body Ptich : Inport  Port=2
  Body Yaw : Inport  Port=3
  WheelFrontLeft Pitch : Inport  Port=4
  WheelFrontRight Pitch : Inport  Port=5
  WheelRearLeft Pitch : Inport  Port=6
  WheelRearRight Ptich : Inport  Port=7
  WheelFrontLeft Roll : Inport  Port=8
  WheelFrontRight Roll : Inport  Port=9
  WheelRearLeft Roll : Inport  Port=10
  WheelRearRight Roll : Inport  Port=11
  WheelFrontLeft Yaw : Inport  Port=12
  WheelFrontRight Yaw : Inport  Port=13
  WheelRearLeft Yaw : Inport  Port=14
  WheelRearRight Yaw : Inport  Port=15
  AllParts : Concatenate  NumInputs=5  Mode=Multidimensional array
  Body : Concatenate  NumInputs=3  Mode=Multidimensional array  ConcatenateDimension=2
  WheelFrontLeft : Concatenate  NumInputs=3  Mode=Multidimensional array  ConcatenateDimension=2
  WheelFrontRight : Concatenate  NumInputs=3  Mode=Multidimensional array  ConcatenateDimension=2
  WheelRearLeft : Concatenate  NumInputs=3  Mode=Multidimensional array  ConcatenateDimension=2
  WheelRearRight : Concatenate  NumInputs=3  Mode=Multidimensional array  ConcatenateDimension=2
  ConcatOut : Outport  VectorParamsAs1DForOutWhenUnconnected=off
  wires:
  Body Yaw/1 -> Body/3
  WheelFrontLeft Yaw/1 -> WheelFrontLeft/3
  WheelFrontLeft/1 -> AllParts/2
  Body/1 -> AllParts/1
  WheelRearLeft/1 -> AllParts/4
  WheelFrontRight/1 -> AllParts/3
  WheelRearRight Yaw/1 -> WheelRearRight/3
  WheelRearLeft Yaw/1 -> WheelRearLeft/3
  AllParts/1 -> ConcatOut/1
  WheelRearRight/1 -> AllParts/5
  WheelFrontRight Yaw/1 -> WheelFrontRight/3
  Body Roll/1 -> Body/1
  Body Ptich/1 -> Body/2
  WheelFrontLeft Pitch/1 -> WheelFrontLeft/2
  WheelFrontLeft Roll/1 -> WheelFrontLeft/1
  WheelFrontRight Roll/1 -> WheelFrontRight/1
  WheelFrontRight Pitch/1 -> WheelFrontRight/2
  WheelRearLeft Roll/1 -> WheelRearLeft/1
  WheelRearLeft Pitch/1 -> WheelRearLeft/2
  WheelRearRight Roll/1 -> WheelRearRight/1
  WheelRearRight Ptich/1 -> WheelRearRight/2

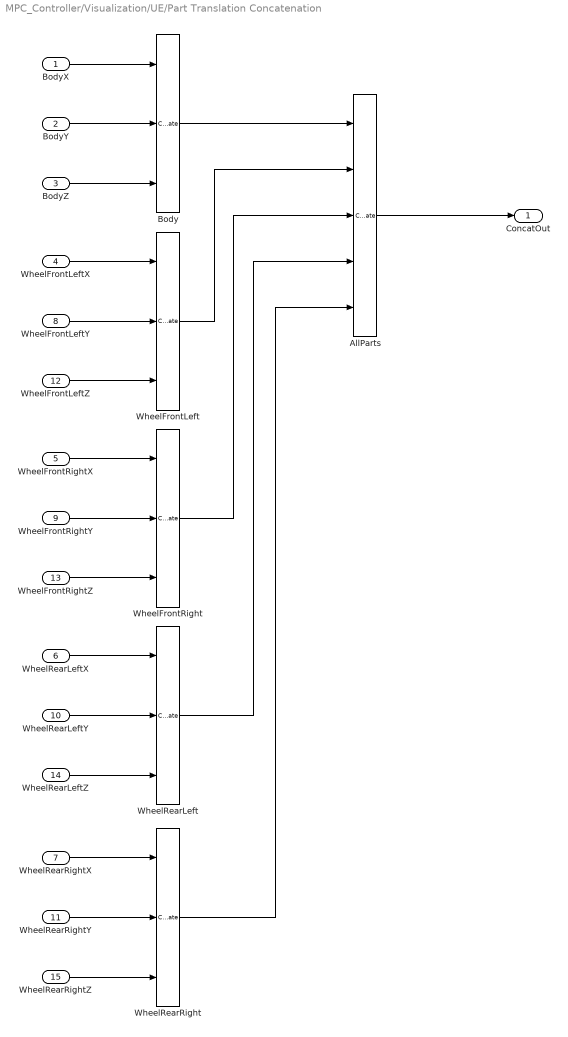
== system MPC_Controller/Visualization/UE/Part Translation Concatenation ==
  BodyX : Inport
  BodyY : Inport  Port=2
  BodyZ : Inport  Port=3
  WheelFrontLeftX : Inport  Port=4
  WheelFrontRightX : Inport  Port=5
  WheelRearLeftX : Inport  Port=6
  WheelRearRightX : Inport  Port=7
  WheelFrontLeftY : Inport  Port=8
  WheelFrontRightY : Inport  Port=9
  WheelRearLeftY : Inport  Port=10
  WheelRearRightY : Inport  Port=11
  WheelFrontLeftZ : Inport  Port=12
  WheelFrontRightZ : Inport  Port=13
  WheelRearLeftZ : Inport  Port=14
  WheelRearRightZ : Inport  Port=15
  AllParts : Concatenate  NumInputs=5  Mode=Multidimensional array
  Body : Concatenate  NumInputs=3  Mode=Multidimensional array  ConcatenateDimension=2
  WheelFrontLeft : Concatenate  NumInputs=3  Mode=Multidimensional array  ConcatenateDimension=2
  WheelFrontRight : Concatenate  NumInputs=3  Mode=Multidimensional array  ConcatenateDimension=2
  WheelRearLeft : Concatenate  NumInputs=3  Mode=Multidimensional array  ConcatenateDimension=2
  WheelRearRight : Concatenate  NumInputs=3  Mode=Multidimensional array  ConcatenateDimension=2
  ConcatOut : Outport  VectorParamsAs1DForOutWhenUnconnected=off
  wires:
  BodyX/1 -> Body/1
  BodyZ/1 -> Body/3
  WheelFrontLeftX/1 -> WheelFrontLeft/1
  WheelFrontLeftZ/1 -> WheelFrontLeft/3
  WheelFrontLeftY/1 -> WheelFrontLeft/2
  BodyY/1 -> Body/2
  WheelFrontLeft/1 -> AllParts/2
  WheelRearRightX/1 -> WheelRearRight/1
  Body/1 -> AllParts/1
  WheelRearLeft/1 -> AllParts/4
  WheelFrontRight/1 -> AllParts/3
  WheelRearRightZ/1 -> WheelRearRight/3
  WheelFrontRightY/1 -> WheelFrontRight/2
  WheelFrontRightX/1 -> WheelFrontRight/1
  WheelRearRightY/1 -> WheelRearRight/2
  WheelRearLeftZ/1 -> WheelRearLeft/3
  AllParts/1 -> ConcatOut/1
  WheelRearLeftY/1 -> WheelRearLeft/2
  WheelRearRight/1 -> AllParts/5
  WheelRearLeftX/1 -> WheelRearLeft/1
  WheelFrontRightZ/1 -> WheelFrontRight/3

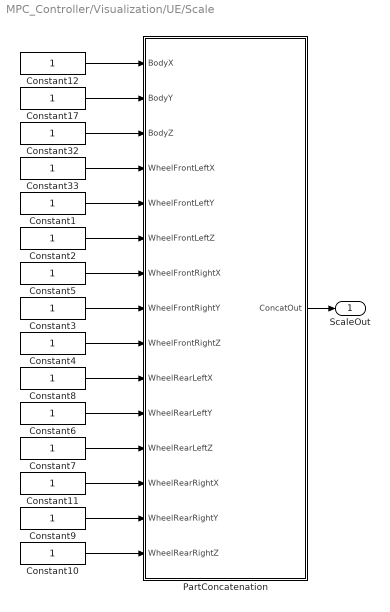
== system MPC_Controller/Visualization/UE/Scale ==
  Constant{1..12,17,32..33} (15 alike) : Constant  OutDataTypeStr=single
  PartConcatenation : Subsystem
  ScaleOut : Outport  VectorParamsAs1DForOutWhenUnconnected=off
  wires:
  Constant10/1 -> PartConcatenation/15(WheelRearRightZ)
  Constant9/1 -> PartConcatenation/14(WheelRearRightY)
  Constant11/1 -> PartConcatenation/13(WheelRearRightX)
  Constant7/1 -> PartConcatenation/12(WheelRearLeftZ)
  Constant6/1 -> PartConcatenation/11(WheelRearLeftY)
  Constant8/1 -> PartConcatenation/10(WheelRearLeftX)
  Constant4/1 -> PartConcatenation/9(WheelFrontRightZ)
  Constant3/1 -> PartConcatenation/8(WheelFrontRightY)
  Constant5/1 -> PartConcatenation/7(WheelFrontRightX)
  Constant2/1 -> PartConcatenation/6(WheelFrontLeftZ)
  Constant1/1 -> PartConcatenation/5(WheelFrontLeftY)
  Constant33/1 -> PartConcatenation/4(WheelFrontLeftX)
  Constant32/1 -> PartConcatenation/3(BodyZ)
  Constant17/1 -> PartConcatenation/2(BodyY)
  Constant12/1 -> PartConcatenation/1(BodyX)
  PartConcatenation/1(ConcatOut) -> ScaleOut/1

== system MPC_Controller/Visualization/Visualization/Vehicle XY Plotter ==
  InertXYZ : Inport
  InertAng : Inport  Port=2
  InertXdotYdotZdot : Inport  Port=3
  WhlAng : Inport  Port=4
  RefXYZ : Inport  Port=5
  Rate Transition{1..5} (5 alike) : RateTransition  Deterministic=off  OutPortSampleTime=Ts
  Vehicle XY Plotter : vehdynlibviscommon/Vehicle XY Plotter  bufferSize=bufferSize  w=w  a=a  b=b  figBorder=figBorder
      settings: SourceProductName=Vehicle Dynamics Blockset  SourceProductBaseCode=VE
  wires:
  InertAng/1 -> Rate Transition2/1  "InertCGDisp"
  InertXdotYdotZdot/1 -> Rate Transition4/1  "InertCGVel"
  InertXYZ/1 -> Rate Transition1/1  "InertCGDisp"
  WhlAng/1 -> Rate Transition5/1  "WhlAng"
  Rate Transition3/1 -> Vehicle XY Plotter/5
  Rate Transition1/1 -> Vehicle XY Plotter/1
  Rate Transition2/1 -> Vehicle XY Plotter/2
  Rate Transition4/1 -> Vehicle XY Plotter/3
  Rate Transition5/1 -> Vehicle XY Plotter/4
  RefXYZ/1 -> Rate Transition3/1

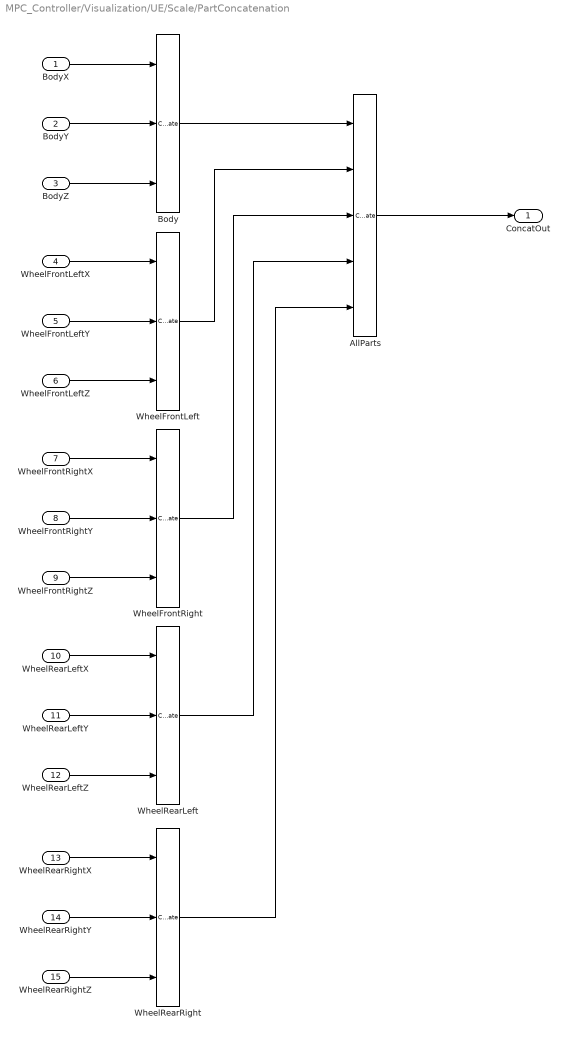
== system MPC_Controller/Visualization/UE/Scale/PartConcatenation ==
  BodyX : Inport
  BodyY : Inport  Port=2
  BodyZ : Inport  Port=3
  WheelFrontLeftX : Inport  Port=4
  WheelFrontLeftY : Inport  Port=5
  WheelFrontLeftZ : Inport  Port=6
  WheelFrontRightX : Inport  Port=7
  WheelFrontRightY : Inport  Port=8
  WheelFrontRightZ : Inport  Port=9
  WheelRearLeftX : Inport  Port=10
  WheelRearLeftY : Inport  Port=11
  WheelRearLeftZ : Inport  Port=12
  WheelRearRightX : Inport  Port=13
  WheelRearRightY : Inport  Port=14
  WheelRearRightZ : Inport  Port=15
  AllParts : Concatenate  NumInputs=5  Mode=Multidimensional array
  Body : Concatenate  NumInputs=3  Mode=Multidimensional array  ConcatenateDimension=2
  WheelFrontLeft : Concatenate  NumInputs=3  Mode=Multidimensional array  ConcatenateDimension=2
  WheelFrontRight : Concatenate  NumInputs=3  Mode=Multidimensional array  ConcatenateDimension=2
  WheelRearLeft : Concatenate  NumInputs=3  Mode=Multidimensional array  ConcatenateDimension=2
  WheelRearRight : Concatenate  NumInputs=3  Mode=Multidimensional array  ConcatenateDimension=2
  ConcatOut : Outport  VectorParamsAs1DForOutWhenUnconnected=off
  wires:
  BodyX/1 -> Body/1
  BodyZ/1 -> Body/3
  WheelFrontLeftX/1 -> WheelFrontLeft/1
  WheelFrontLeftZ/1 -> WheelFrontLeft/3
  WheelFrontLeftY/1 -> WheelFrontLeft/2
  BodyY/1 -> Body/2
  WheelFrontLeft/1 -> AllParts/2
  WheelRearRightX/1 -> WheelRearRight/1
  Body/1 -> AllParts/1
  WheelRearLeft/1 -> AllParts/4
  WheelFrontRight/1 -> AllParts/3
  WheelRearRightZ/1 -> WheelRearRight/3
  WheelFrontRightY/1 -> WheelFrontRight/2
  WheelFrontRightX/1 -> WheelFrontRight/1
  WheelRearRightY/1 -> WheelRearRight/2
  WheelRearLeftZ/1 -> WheelRearLeft/3
  AllParts/1 -> ConcatOut/1
  WheelRearLeftY/1 -> WheelRearLeft/2
  WheelRearRight/1 -> AllParts/5
  WheelRearLeftX/1 -> WheelRearLeft/1
  WheelFrontRightZ/1 -> WheelFrontRight/3

== matlab function MPC_Controller/Scenario Reader/Pack Ego Actor1 ==
  data: pos input; a output Bus: BusActors2Actors size=1; vel input; yaw input; yawRate input
function a = packEgo(pos,vel,yaw,yawRate)
% Pack ego information into a single ego actor bus
%
% Imoprtant note:
% Output is a bus of type BusActorsActors. This is the same bus used by the
% Scenario Reader to output an individual actor. If you change the
% output bus name of Scenario Reader change the output bus name here
% as well by clicking on 'Edit Data' in the menu above.

a = struct(...
    'ActorID',1,...
    'Position', [pos(1) pos(2) 0], ...
    'Velocity', [vel(1) vel(2) 0], ...
    'Roll', 0, ...
    'Pitch', 0, ...
    'Yaw', yaw, ...
    'AngularVelocity', [0 0 yawRate]);

== matlab function MPC_Controller/MPC/Lane Center/MATLAB Function ==
  data: lanes input
  events: fcnLeftAndRight output FUNCTION_CALL_EVENT; fcnLeftOnly output FUNCTION_CALL_EVENT; fcnRightOnly output FUNCTION_CALL_EVENT; fcnNone output FUNCTION_CALL_EVENT
function fcn(lanes)

leftStrength  = lanes.Left.Strength;
rightStrength = lanes.Right.Strength;

if (leftStrength > 0) && (rightStrength > 0)
   fcnLeftAndRight();
   
elseif leftStrength > 0
    fcnLeftOnly();
    
elseif rightStrength > 0
    fcnRightOnly();
    
else
    fcnNone();
end

== matlab function MPC_Controller/MPC/Lane Center/Preview Curvature ==
  data: rho output; Curvature0 input; dCurvature input; Vx input; Ts parameter
function rho = predictCurvature(Curvature0,dCurvature,Vx, Ts)
% Curvature0 = initial curvature per unit length                  [1/m]
% dCurvature = (constant) derivative of curvature per unit length [1/m^2]
% CurvatureLength = length for which the clothoid model is valid [m]
% Vx = speed of vehicle

% We want to export a set of curvatures at a uniform sample time ahead.
% t is this vector which goes up to 1 second in the future or having
% enough time to reach the known length in curvature (whichever is smaller)

% To enable truncation by curvelength, mark output "rho" as varsize
%t = 0:Ts:min(1,CurvatureLength/Vx);

t = zeros(10+1,1);
for i=1:numel(t)
    t(i) = (i-1).*Ts;
end

% We compute the curvature vector rho(t) using the specified clothoid model
rho = Curvature0 + dCurvature*Vx*t;
